simulink model "kocenje"  (R2017b)
settings: Solver=VariableStepAuto  StartTime=0.0  StopTime=10.0  RelTol=1e-3
libraries: fuzblock x1
settings Model: Creator=DT User  LastModifiedBy=DT User

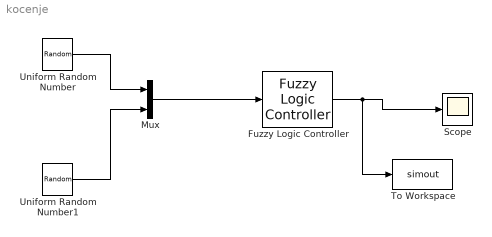
== system kocenje ==
  Fuzzy Logic Controller : fuzblock/Fuzzy Logic  Controller  FIS=kocenje  OutputSampleNumber=101  DataType=double  FuzzifiedInputs=off  RuleFiringStrengths=off  RuleOutputs=off  AggregatedOutputs=off  SimulateUsing=Interpreted execution
  Mux : Mux  Inputs=2
  Scope : Scope
  To Workspace : ToWorkspace  VariableName=simout  SaveFormat=Timeseries  SampleTime=-1
  Uniform Random Number : UniformRandomNumber  Minimum=10  Maximum=100  SampleTime=0.1
  Uniform Random Number1 : UniformRandomNumber  Minimum=10  Maximum=150  SampleTime=0.1
  wires:
  Mux/1 -> Fuzzy Logic Controller/1
  Uniform Random Number/1 -> Mux/1
  Uniform Random Number1/1 -> Mux/2
  Fuzzy Logic Controller/1 -> To Workspace/1, Scope/1
